simulink model "LQR_Gain_Scheduled"  (R2017a)
settings: Solver=FixedStepAuto  StartTime=0.0  StopTime=10  FixedStep=0.0001  RelTol=1e-3
values from neighbouring files (symbols this model uses):
  Cf = 30989    [LQR_Gain_Scheduled_Setup_2017.m]
  Cr = 50154    [LQR_Gain_Scheduled_Setup_2017.m]
  Iz = 111.8    [LQR_Gain_Scheduled_Setup_2017.m]
  lf = 0.783    [LQR_Gain_Scheduled_Setup_2017.m]
  lr = 0.752    [LQR_Gain_Scheduled_Setup_2017.m]
  m = 245    [LQR_Gain_Scheduled_Setup_2017.m]
undefined symbols (not defined in the file or in its folder): DiscIntNeverNeededParam, K1, K2, K3
libraries: dspsrcs4 x3
settings Model: Creator=Johan PC  LastModifiedBy=Johan PC
settings SFSimCC: SimUseLocalCustomCode=on
settings RTWCC: RTWUseLocalCustomCode=on

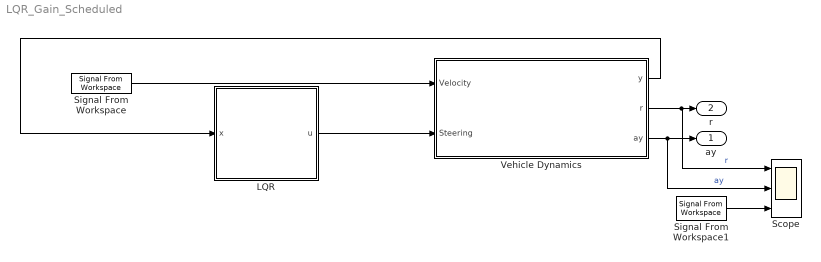
== system LQR_Gain_Scheduled ==
  LQR : Subsystem
  Scope : Scope  NumInputPorts=3
  Signal From Workspace : dspsrcs4/Signal From Workspace  X=Velocity  Ts=0.1  nsamps=1  OutputAfterFinalValue=Setting to zero  ignoreOrWarnInputAndFrameLengths=off  OutputFrames=off
  Signal From Workspace1 : dspsrcs4/Signal From Workspace  X=ref_yalmip  Ts=0.1  nsamps=1  OutputAfterFinalValue=Setting to zero  ignoreOrWarnInputAndFrameLengths=off  OutputFrames=off
  Vehicle Dynamics : Subsystem
  ay : Outport
  r : Outport  Port=2
  wires:
  Vehicle Dynamics/1("y ") -> LQR/1(x)
  LQR/1(u) -> Vehicle Dynamics/2(Steering)
  Signal From Workspace/1 -> Vehicle Dynamics/1(Velocity)
  Vehicle Dynamics/3(ay) -> Scope/2, ay/1  "ay"
  Vehicle Dynamics/2("r ") -> Scope/1, r/1  "r"
  Signal From Workspace1/1 -> Scope/3

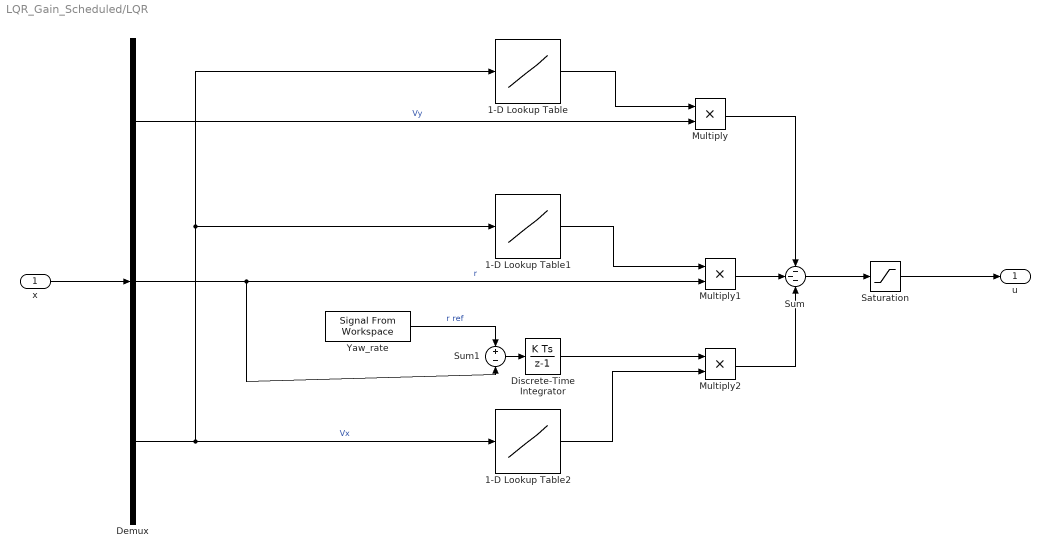
== system LQR_Gain_Scheduled/LQR ==
  x : Inport
  1-D Lookup Table : Lookup_n-D  NumberOfTableDimensions=1  BreakpointsSpecification=Even spacing  BreakpointsForDimension1=[-5:5]  BreakpointsForDimension1FirstPoint=5  BreakpointsForDimension1Spacing=5  Table=K1  InternalRulePriority=Speed  RndMeth=Simplest  InputSameDT=on
  1-D Lookup Table1 : Lookup_n-D  NumberOfTableDimensions=1  BreakpointsSpecification=Even spacing  BreakpointsForDimension1=[-5:5]  BreakpointsForDimension1FirstPoint=5  BreakpointsForDimension1Spacing=5  Table=K2  InternalRulePriority=Speed  RndMeth=Simplest  InputSameDT=on
  1-D Lookup Table2 : Lookup_n-D  NumberOfTableDimensions=1  BreakpointsSpecification=Even spacing  BreakpointsForDimension1=[-5:5]  BreakpointsForDimension1FirstPoint=5  BreakpointsForDimension1Spacing=5  Table=K3  InternalRulePriority=Speed  RndMeth=Simplest  InputSameDT=on
  Demux : Demux  Outputs=3
  Discrete-Time Integrator : DiscreteIntegrator  InitialConditionSetting=State (most efficient)  SampleTime=0.001  ICPrevOutput=DiscIntNeverNeededParam  ICPrevScaledInput=DiscIntNeverNeededParam
  Multiply : Product
  Multiply1 : Product
  Multiply2 : Product
  Saturation : Saturate  UpperLimit=0.45  LowerLimit=-0.45
  Sum : Sum  Inputs=---
  Sum1 : Sum  Inputs=+-
  Yaw_rate : dspsrcs4/Signal From Workspace  X=Yawrate  Ts=0.1  nsamps=1  OutputAfterFinalValue=Setting to zero  ignoreOrWarnInputAndFrameLengths=off  OutputFrames=off
  u : Outport
  wires:
  Discrete-Time Integrator/1 -> Multiply2/1
  Multiply2/1 -> Sum/3
  x/1 -> Demux/1
  Demux/2 -> Multiply1/2, Sum1/2  "r"
  Multiply/1 -> Sum/1
  Multiply1/1 -> Sum/2
  Sum/1 -> Saturation/1
  Sum1/1 -> Discrete-Time Integrator/1
  Yaw_rate/1 -> Sum1/1  "r ref"
  Saturation/1 -> u/1
  1-D Lookup Table/1 -> Multiply/1
  Demux/1 -> Multiply/2  "Vy"
  Demux/3 -> 1-D Lookup Table/1, 1-D Lookup Table1/1, 1-D Lookup Table2/1  "Vx"
  1-D Lookup Table1/1 -> Multiply1/1
  1-D Lookup Table2/1 -> Multiply2/2

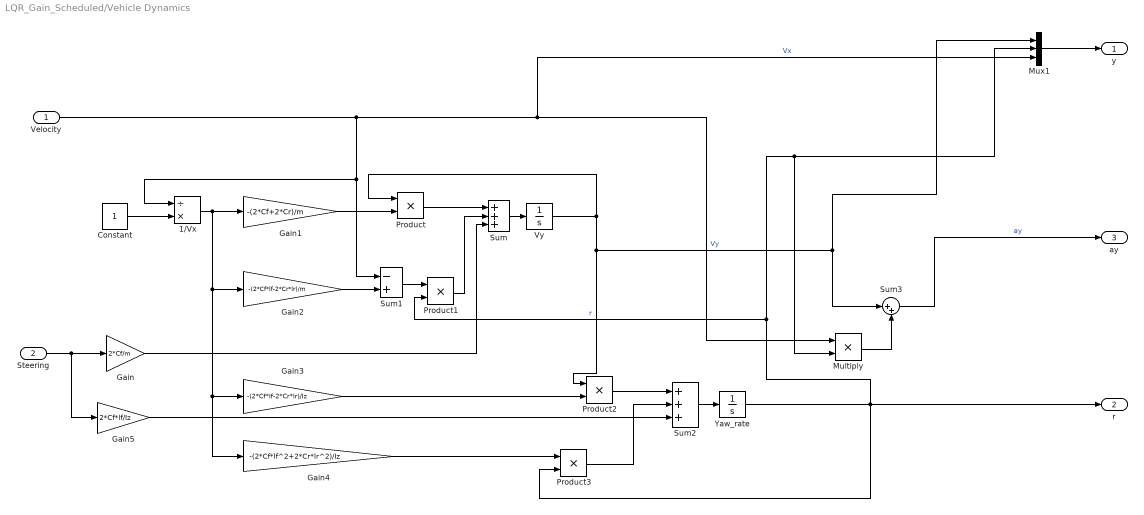
== system LQR_Gain_Scheduled/Vehicle Dynamics ==
  Velocity : Inport
  Steering : Inport  Port=2
  1/Vx : Product  Inputs=/*
  Constant : Constant
  Gain : Gain  Gain=2*Cf/m
  Gain1 : Gain  Gain=-(2*Cf+2*Cr)/m
  Gain2 : Gain  Gain=-(2*Cf*lf-2*Cr*lr)/m
  Gain3 : Gain  Gain=-(2*Cf*lf-2*Cr*lr)/Iz
  Gain4 : Gain  Gain=-(2*Cf*lf^2+2*Cr*lr^2)/Iz
  Gain5 : Gain  Gain=2*Cf*lf/Iz
  Multiply : Product
  Mux1 : Mux  Inputs=3
  Product{,1..3} (4 alike) : Product
  Sum : Sum  Inputs=+++
  Sum1 : Sum  Inputs=-+
  Sum2 : Sum  Inputs=+++
  Sum3 : Sum  Inputs=|++
  Vy : Integrator
  "Yaw_rate " : Integrator
  "y " : Outport
  "r " : Outport  Port=2
  ay : Outport  Port=3
  wires:
  Sum2/1 -> "Yaw_rate "/1
  Gain2/1 -> Sum1/2
  Gain4/1 -> Product3/1
  Constant/1 -> 1/Vx/2
  Gain3/1 -> Product2/2
  1/Vx/1 -> Gain4/1, Gain3/1, Gain2/1, Gain1/1
  Product2/1 -> Sum2/1
  Product3/1 -> Sum2/2
  Gain5/1 -> Sum2/3
  Sum1/1 -> Product1/1
  "Yaw_rate "/1 -> Multiply/2, Mux1/2, Product1/2, "r "/1, Product3/2  "r"
  Gain/1 -> Sum/3
  Steering/1 -> Gain/1, Gain5/1
  Gain1/1 -> Product/2
  Product/1 -> Sum/1
  Vy/1 -> Mux1/1, Sum3/1, Product2/1, Product/1  "Vy"
  Sum/1 -> Vy/1
  Velocity/1 -> Mux1/3, Multiply/1, 1/Vx/1, Sum1/1  "Vx"
  Product1/1 -> Sum/2
  Multiply/1 -> Sum3/2
  Sum3/1 -> ay/1  "ay"
  Mux1/1 -> "y "/1
